simulink model "AERO560_HW6_Sim2_Thapar"  (R2022b)
settings: Solver=VariableStepAuto  StartTime=0.0  StopTime=10.0  RelTol=1e-3
undefined symbols (not defined in the file or in its folder): p2
settings Model: Creator=gagandeepthapar  LastModifiedBy=gagandeepthapar

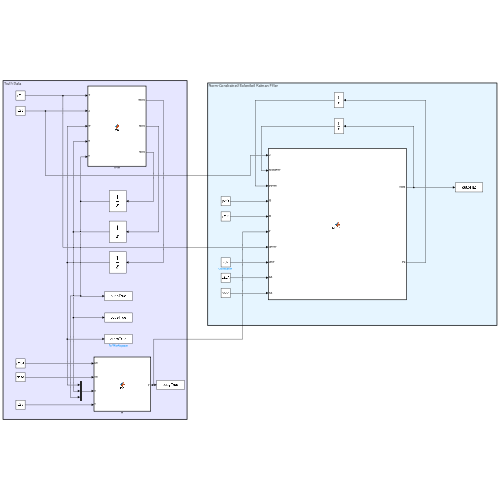
[thumbnail: Simulink's stored preview of the top-level diagram]
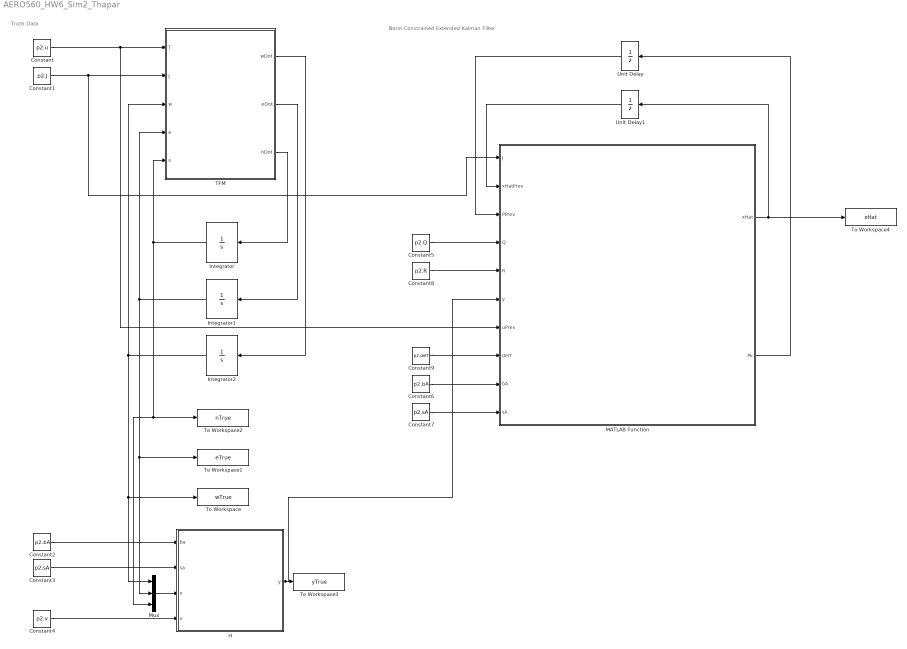
== system AERO560_HW6_Sim2_Thapar ==
  note: Norm-Constrained Extended Kalman Filter
  note: Truth Data
  Constant : Constant  Value=p2.u
  Constant1 : Constant  Value=p2.J
  Constant2 : Constant  Value=p2.bA
  Constant3 : Constant  Value=p2.sA
  Constant4 : Constant  Value=p2.v
  Constant5 : Constant  Value=p2.Q
  Constant6 : Constant  Value=p2.bA
  Constant7 : Constant  Value=p2.sA
  Constant8 : Constant  Value=p2.R
  Constant9 : Constant  Value=p2.delT
  H : MATLAB Function  TreatAsAtomicUnit=on
  Integrator : Integrator  InitialCondition=p2.n0
  Integrator1 : Integrator  InitialCondition=p2.e0
  Integrator2 : Integrator  InitialCondition=p2.w0
  MATLAB Function : MATLAB Function  TreatAsAtomicUnit=on
  Mux : Mux  Inputs=3
  TFM : MATLAB Function  TreatAsAtomicUnit=on
  To Workspace : ToWorkspace  VariableName=wTrue  SampleTime=-1
      settings: Save2DSignal=2-D array (concatenate along first dimension)
  To Workspace1 : ToWorkspace  VariableName=eTrue  SampleTime=-1
      settings: Save2DSignal=2-D array (concatenate along first dimension)
  To Workspace2 : ToWorkspace  VariableName=nTrue  SampleTime=-1
      settings: Save2DSignal=2-D array (concatenate along first dimension)
  To Workspace3 : ToWorkspace  VariableName=yTrue  SampleTime=-1
      settings: Save2DSignal=2-D array (concatenate along first dimension)
  To Workspace4 : ToWorkspace  VariableName=xHat  SampleTime=-1
      settings: Save2DSignal=2-D array (concatenate along first dimension)
  Unit Delay : UnitDelay  InitialCondition=p2.Pk0  SampleTime=-1  HasFrameUpgradeWarning=on
  Unit Delay1 : UnitDelay  InitialCondition=[p2.wHat0;p2.eHat0;p2.nHat0]  SampleTime=-1  HasFrameUpgradeWarning=on
  wires:
  TFM/1(wDot) -> Integrator2/1
  TFM/2(eDot) -> Integrator1/1
  TFM/3(nDot) -> Integrator/1
  Integrator/1 -> TFM/5(n), Mux/3, To Workspace2/1
  Integrator1/1 -> Mux/2, To Workspace1/1, TFM/4(e)
  Integrator2/1 -> TFM/3(w), Mux/1, To Workspace/1
  Constant/1 -> MATLAB Function/7(uPrev), TFM/1(T)
  Constant1/1 -> MATLAB Function/1(J), TFM/2(J)
  Constant2/1 -> H/1(ba)
  Constant3/1 -> H/2(sa)
  Constant4/1 -> H/4(v)
  H/1(y) -> MATLAB Function/6(y), To Workspace3/1
  Mux/1 -> H/3(x)
  MATLAB Function/2(Pk) -> Unit Delay/1
  MATLAB Function/1(xHat) -> To Workspace4/1, Unit Delay1/1
  Unit Delay1/1 -> MATLAB Function/2(xHatPrev)
  Unit Delay/1 -> MATLAB Function/3(PPrev)
  Constant5/1 -> MATLAB Function/4(Q)
  Constant8/1 -> MATLAB Function/5(R)
  Constant9/1 -> MATLAB Function/8(delT)
  Constant7/1 -> MATLAB Function/10(sA)
  Constant6/1 -> MATLAB Function/9(bA)

== matlab function AERO560_HW6_Sim2_Thapar/H ==
  data: ba input; y output; sa input; x input; v input
function y = fcn(ba, sa, x, v)
    
    function wx = skewSymmetric(w)
        wx = [0, -1*w(3), w(2);
             w(3), 0, -1*w(1);
             -1*w(2), w(1), 0];
    end

    
    function Yaq = Y_aa_q(a, e, n)

        Ya = [n*eye(3)-skewSymmetric(e), -e];
        Yb = [skewSymmetric(a), a; -a', 0];
        Yaq = Ya*Yb;
        
    end

e = x(4:6);
n = x(7);

y = [zeros(3,3), Y_aa_q(ba, e, n);
     zeros(3,3), Y_aa_q(sa, e, n)] * x + v;

end

== matlab function AERO560_HW6_Sim2_Thapar/TFM ==
  data: T input; J input; w input; e input; n input; wDot output; eDot output; nDot output
function [wDot, eDot, nDot] = fcn(T, J, w, e, n)
    
    function wx = skewSymmetric(w)
        wx = [0, -1*w(3), w(2);
             w(3), 0, -1*w(1);
             -1*w(2), w(1), 0];
    end

wDot = J\(T-skewSymmetric(w)*J*w);

eDot = 0.5*(n*eye(3) + skewSymmetric(e))*w;
nDot = -0.5*e'*w;

end

== matlab function AERO560_HW6_Sim2_Thapar/MATLAB Function ==
  data: xHat output; J input; xHatPrev input; PPrev input; Q input; R input; y input; uPrev input; delT input; Pk output; bA input; sA input
function [xHat, Pk] = NCEKF(J, xHatPrev, PPrev, Q, R, y, uPrev, delT, bA, sA)
    
    function wx = skewSymmetric(w)
        wx = [0, -1*w(3), w(2);
             w(3), 0, -1*w(1);
             -1*w(2), w(1), 0];
    end

    function Yaq = Y_aa_q(a, e, n)

        Ya = [n*eye(3)-skewSymmetric(e), -e];
        Yb = [skewSymmetric(a), a; -a', 0];
        Yaq = Ya*Yb;
        
    end

    function dstate = TFM(state, T, J)

        w = state(1:3);
        e = state(4:6);
        n = state(7);

        wDot = J\(T-skewSymmetric(w)*J*w);
        
        eDot = 0.5*(n*eye(3) + skewSymmetric(e))*w;
        nDot = -0.5*e'*w;

        dstate = [wDot;eDot;nDot];
    end

% predictor
wHatPrev = [xHatPrev(1);xHatPrev(2);xHatPrev(3)];
eHatPrev = [xHatPrev(4);xHatPrev(5);xHatPrev(6)];
nHatPrev = xHatPrev(7);

rowA = [J\(-skewSymmetric(wHatPrev)*J + skewSymmetric(J*wHatPrev)), zeros(3,3), zeros(3,1)];
rowB = [0.5*(nHatPrev*eye(3) + skewSymmetric(eHatPrev)), -0.5*skewSymmetric(wHatPrev), 0.5*wHatPrev];
rowC = [-0.5*eHatPrev', -0.5*wHatPrev', 0];

FPrev = eye(7) + delT * [rowA;rowB;rowC];
LPrev = [delT*inv(J);zeros(3,3);zeros(1,3)];

f_hat_prev = TFM([wHatPrev;eHatPrev;nHatPrev], uPrev, J);

xHatMinus = xHatPrev + f_hat_prev*delT;
wHatMinus = xHatMinus(1:3);
eHatMinus = xHatMinus(4:6);
nHatMinus = xHatMinus(7);

PkMinus = FPrev*PPrev*FPrev' + LPrev*Q*LPrev';

PkMinus_1 = PkMinus(:,1:3);
PkMinus_2 = PkMinus(:,4:7);

PkMinus_ww = PkMinus(1:3,1:3);
PkMinus_qw = PkMinus(4:7,1:3);
PkMinus_wq = PkMinus(1:3,4:7);
PkMinus_qq = PkMinus(4:7,4:7);

% corrector
M = eye(6);
H = [zeros(3,3), Y_aa_q(bA, eHatMinus, nHatMinus);
       zeros(3,3), Y_aa_q(sA, eHatMinus, nHatMinus)];

W = H*PkMinus*H' + M*R*M';
K_w = PkMinus_1'*H'*inv(W);
h_y = H*xHatMinus;
wHat = wHatMinus + K_w*(y - h_y);

K_tilde = PkMinus_2'*H'*inv(W);
r_k_vec = y - h_y;
r_k_scl = r_k_vec'*inv(W)*r_k_vec;

q_tilde = [eHatMinus;nHatMinus] + K_tilde*r_k_vec;

K_qk = K_tilde + 1/r_k_scl * (1/norm(q_tilde) - 1)*q_tilde*r_k_vec'*inv(W);

qHat = [eHatMinus;nHatMinus] + K_qk*r_k_vec;

xHat = [wHat;qHat];

Pk_ww = PkMinus_ww - K_w*H*PkMinus_1 - PkMinus_1'*H'*K_w' + K_w*W*K_w';
Pk_wq = PkMinus_wq - K_w*H*PkMinus_2 - PkMinus_1'*H'*K_qk' + K_w*W*K_qk';
Pk_qw = PkMinus_qw - K_qk*H*PkMinus_1 - PkMinus_2'*H'*K_w' + K_qk*W*K_w';
Pk_qq = PkMinus_qq - K_qk*H*PkMinus_2 - PkMinus_2'*H'*K_qk' + K_qk*W*K_qk';

Pk = [Pk_ww, Pk_wq; Pk_qw, Pk_qq];

end
